simulink library "VectorLibrary"  (R2015a)
settings: Solver=ode45  StartTime=0.0  StopTime=10.0  RelTol=1e-3
settings Model: Creator=Cam  LastModifiedBy=Cam

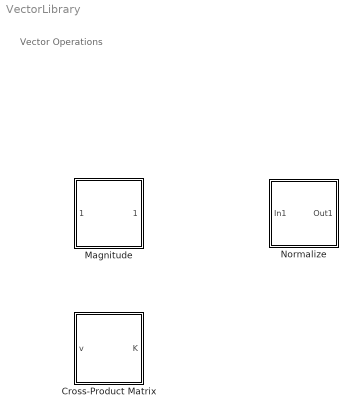
== system VectorLibrary ==
  note: Vector Operations
  Cross-Product Matrix : Subsystem  mask(Cross-Product Matrix){}
      mask help: Converts a 3x1 vector into its cross-product matrix.
      mask Display: disp('v \rightarrow V^\times','texmode','on')
  Magnitude : Subsystem  mask(Magnitude){}
      mask help: Returns the magnitude of the given vector.
      mask Display: disp('||u||', 'texmode','on')
  Normalize : Subsystem  mask(Normalize){}
      mask help: Normalizes the given vector.
      mask Display: disp('u / ||u||', 'texmode','on')

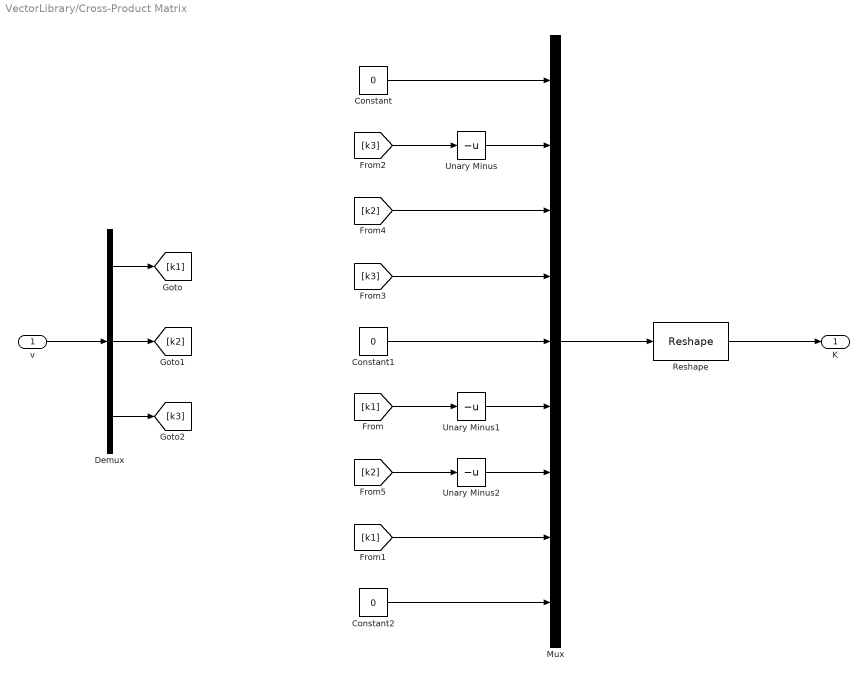
== system VectorLibrary/Cross-Product Matrix ==
  v : Inport
  Constant : Constant  Value=0
  Constant1 : Constant  Value=0
  Constant2 : Constant  Value=0
  Demux : Demux  Outputs=3
  Mux : Mux  Inputs=9
  Reshape : Reshape  OutputDimensionality=Customize  OutputDimensions=[3,3]
  Unary Minus : UnaryMinus
  Unary Minus1 : UnaryMinus
  Unary Minus2 : UnaryMinus
  K : Outport
  wires:
  v/1 -> Demux/1
  Reshape/1 -> K/1
  Mux/1 -> Reshape/1
  Unary Minus1/1 -> Mux/6
  Unary Minus/1 -> Mux/2
  Unary Minus2/1 -> Mux/7
  Demux/3 -> [k3]
  Demux/2 -> [k2]
  Demux/1 -> [k1]
  [k1] -> Unary Minus1/1
  [k1] -> Mux/8
  [k3] -> Unary Minus/1
  [k3] -> Mux/4
  Constant/1 -> Mux/1
  Constant2/1 -> Mux/9
  Constant1/1 -> Mux/5
  [k2] -> Mux/3
  [k2] -> Unary Minus2/1

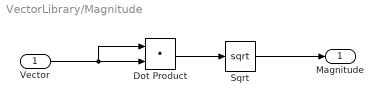
== system VectorLibrary/Magnitude ==
  Vector : Inport
  Dot Product : DotProduct  InputSameDT=on  OutDataTypeStr=Inherit: Inherit via internal rule
  Sqrt : Sqrt  SaturateOnIntegerOverflow=on
  Magnitude : Outport
  wires:
  Dot Product/1 -> Sqrt/1
  Sqrt/1 -> Magnitude/1
  Vector/1 -> Dot Product/2, Dot Product/1

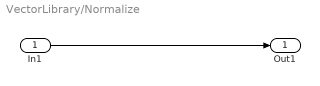
== system VectorLibrary/Normalize ==
  In1 : Inport
  Out1 : Outport
  wires:
  In1/1 -> Out1/1
